simulink model "FinalModel"  (R2017b)
settings: Solver=VariableStepAuto  StartTime=0.0  StopTime=0.1  MaxStep=1e-4  RelTol=1e-3
undefined symbols (not defined in the file): D1, Delta
libraries: powerlib x31, powerlib_meascontrol x9, simulink x1, re_lib x1
settings Model: Creator=User1  LastModifiedBy=User1

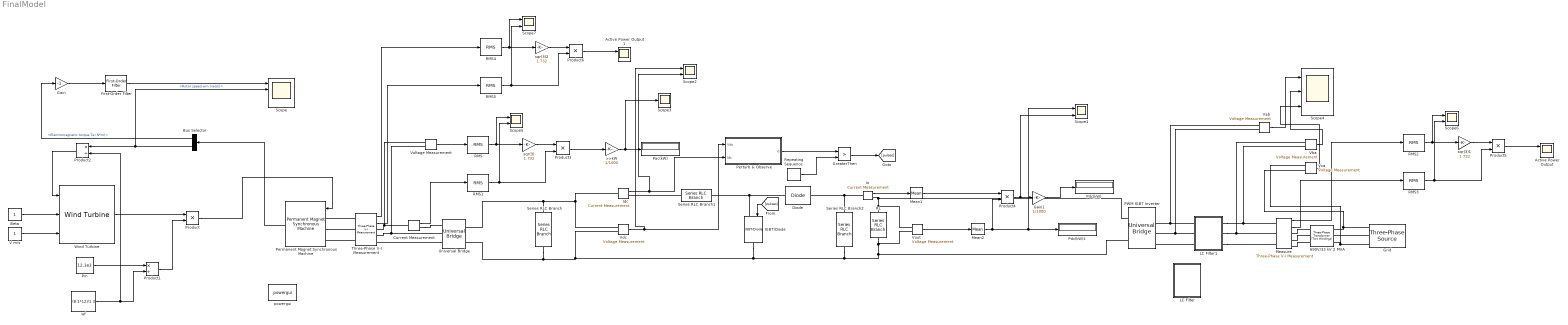
== system FinalModel ==
  690V/33 kV 2 MVA : powerlib/Elements/Three-Phase Transformer (Two Windings)  Winding1Connection=Yg  Winding2Connection=Delta (D1)  CoreType=Three single-phase transformers  SetSaturation=off  Hysteresis=off  DataFile='basic_model'  SetInitialFlux=off  Measurements=None  UNITS=SI  NominalPower=[2e6 50 ]  Winding1=[690 0.0006348 6.0619e-05]  Winding2=[33000 4.356 0.41597]  Rm=119.03  Lm=0.37887  L0=0.5  Saturation=[0 0;11.833 2.152;2366.7 2.5106]  InitialFluxes=[1.4346 -1.4346 1.2553]  MoreParameters=off  BreakLoop=off  DataType=on  TransfoNumber=0
  >>kW : Gain  Gain=1/1000
  "Active Power Output " : Scope  NumInputPorts=2
  Active Power Output 1 : Scope  NumInputPorts=2
  Beta : Constant
  Bus Selector : BusSelector  OutputSignals=Electromagnetic torque Te (N*m),Rotor speed wm (rad/s)
  Current Measurement : powerlib/Measurements/Current Measurement  PhasorSimulation=off  OutputType=Complex  PSBequivalent=0
  Diode : powerlib/Power Electronics/Diode  Ron=0.001  Lon=0  Vf=0.8  IC=0  UseSnubber=0  Rs=inf  Cs=inf  Measurements=off
  First-Order Filter : powerlib_meascontrol/Filters/First-Order Filter  FilterType=Lowpass  Tc=10e-3  Ts=50e-6  Initialize=on  Vac_Init=[0, 0, 50]  Vdc_Init=0  PlotResponse=off  FreqRange="[0,  200,  1]"
      settings: SourceProductName=Simscape Power Systems
  Gain : Gain  Gain=-1
  Gain1 : Gain  Gain=1/1000
  GreaterThen : RelationalOperator  Operator=>  OutDataTypeStr=boolean  RndMeth=Simplest
  Grid : powerlib/Electrical Sources/Three-Phase Source  InternalConnection=Yg  VoltagePhases=off  Voltage=19052  PhaseAngle=0  Voltage_phases=[25e3 25e3 25e3]/sqrt(3)  PhaseAngles_phases=[0 -120 +120]  Frequency=50  NonIdealSource=on  SpecifyImpedance=on  Resistance=0.8929  Inductance=16.58e-3  ShortCircuitLevel=2e6  BaseVoltage=33e3  XRratio=7  BusType=swing  Pref=10e3  Qref=0  Prefabc=[10e3, 10e3, 10e3]  Qrefabc=[0, 0, 0]  Qmin=-inf  Qmax=inf
  IGBT/Diode : powerlib/Power Electronics/IGBT//Diode  Ron=1e-3  Rs=1e5  Cs=inf  Measurements=off
  Idc : powerlib/Measurements/Current Measurement  PhasorSimulation=off  OutputType=Complex  PSBequivalent=0
  Io : powerlib/Measurements/Current Measurement  PhasorSimulation=off  OutputType=Complex  PSBequivalent=0
  LC Filter : Subsystem
  LC Filter1 : Subsystem
  Mean1 : powerlib_meascontrol/Measurements/Mean  Freq=60  Vinit=0  Ts=0
  Mean2 : powerlib_meascontrol/Measurements/Mean  Freq=60  Vinit=0  Ts=0
  Measure : powerlib/Measurements/Three-Phase V-I Measurement  VoltageMeasurement=phase-to-ground  SetLabelV=off  LabelV=V1  Vpu=off  VpuLL=off  CurrentMeasurement=yes  SetLabelI=off  LabelI=I1  Ipu=off  Pbase=1e3  Vbase=380  OutputType=Magnitude  PhasorSimulation=off  PSBequivalent=0
  PWM IGBT Inverter : powerlib/Power Electronics/Universal Bridge  Arms=3  SnubberResistance=5000  SnubberCapacitance=inf  Device=IGBT / Diodes  Ron=1e-3  Lon=0  ForwardVoltages="[  0.0  0.0  ]"  ForwardVoltage=.8  GTOparameters=[ 1e-6 ,1e-6 ]  IGBTparameters=[ 1e-6 , 2e-6 ]  Measurements=All voltages and currents  Measurements_2=None  converterType=Rectifier
  Pac(kW) : Display
  Pdc(kW) : Display
  Pdc(kW)1 : Display
  Permanent Magnet Synchronous Machine : powerlib/Machines/Permanent Magnet Synchronous Machine  NbPhases=3  FluxDistribution=Sinusoidal  RotorType=Salient-pole  MechanicalLoad=Torque Tm  PresetModel=No  ShowDetailedParameters=on  MeasurementBus=off  Resistance=0.00485  Inductance=8.5e-3  dqInductances=[0.295e-3,0.395e-3]  La=0.000835  MachineConstant=Voltage Constant (V_peak L-L / krpm)  Flux=0.77186  VoltageCst=700  TorqueCst=5.789  Flat=120  Mechanical=[0.00062 0.0003035 5 0]  PolePairs=5  InitialConditions=[0,0, 0,0]  InitialConditions5ph=[0 0 0 0 0 0]  TsPowergui=0  TsBlock=-1  RefAngle=90 degrees behind phase A axis (modified Park)
      settings: SourceProductName=Simscape Power Systems
  Perturb & Observe : Subsystem
  Pm : Constant  Value=12.3e3
  Product : Product  Inputs=**
  Product1 : Product  Inputs=*/
  Product2 : Product  Inputs=*/
  Product{3..6} (4 alike) : Product
  RL : powerlib/Elements/Series RLC Branch  LConnTagsString=__new0  RConnTagsString=__new0  BranchType=R  Resistance=0.2380  Inductance=1e-3  SetiL0=off  InitialCurrent=0  Capacitance=500e-6  Setx0=off  InitialVoltage=0  Measurements=None
  RMS : powerlib_meascontrol/Measurements/RMS  TrueRMS=on  Freq=50  RMSInit=650  Ts=0.1
  RMS1 : powerlib_meascontrol/Measurements/RMS  TrueRMS=on  Freq=50  RMSInit=650  Ts=0.1
  RMS{2..5} (4 alike) : powerlib_meascontrol/Measurements/RMS  TrueRMS=on  Freq=50  RMSInit=690  Ts=0.1
  Repeating Sequence : simulink/Sources/Repeating Sequence  rep_seq_t=[0 1/20000]  rep_seq_y=[0 0.9]
  Scope : Scope  NumInputPorts=4
  Scope{1..2,5..7} (5 alike) : Scope  NumInputPorts=2
  Scope3 : Scope
  Scope4 : Scope  NumInputPorts=3
  Series RLC Branch : powerlib/Elements/Series RLC Branch  LConnTagsString=__new0  RConnTagsString=__new0  BranchType=RC  Resistance=0.005  Inductance=1e-3  SetiL0=off  InitialCurrent=0  Capacitance=500e-6  Setx0=off  InitialVoltage=0  Measurements=None
  Series RLC Branch1 : powerlib/Elements/Series RLC Branch  LConnTagsString=__new0  RConnTagsString=__new0  BranchType=L  Resistance=0  Inductance=6.123e-06  SetiL0=off  InitialCurrent=0  Capacitance=1e-6  Setx0=off  InitialVoltage=0  Measurements=None
  Series RLC Branch2 : powerlib/Elements/Series RLC Branch  LConnTagsString=__new0  RConnTagsString=__new0  BranchType=RC  Resistance=0.005  Inductance=1e-3  SetiL0=off  InitialCurrent=0  Capacitance=0.0088  Setx0=off  InitialVoltage=0  Measurements=None
  Three-Phase V-I Measurement : powerlib/Measurements/Three-Phase V-I Measurement  VoltageMeasurement=phase-to-phase  SetLabelV=off  LabelV=Vabc  Vpu=off  VpuLL=off  CurrentMeasurement=yes  SetLabelI=off  LabelI=Iabc  Ipu=off  Pbase=100e6  Vbase=500e3  OutputType=Complex  PhasorSimulation=off  PSBequivalent=0
  Universal Bridge : powerlib/Power Electronics/Universal Bridge  Arms=3  SnubberResistance=1e5  SnubberCapacitance=inf  Device=Diodes  Ron=1e-3  Lon=0  ForwardVoltages="[  0  0  ]"  ForwardVoltage=0  GTOparameters=[ 10e-6 , 20e-6 ]  IGBTparameters=[ 1e-6 , 2e-6 ]  Measurements=None  Measurements_2=None  converterType=Rectifier
  V m/s : Constant
  Vab : powerlib/Measurements/Voltage Measurement  Tag=PoWeRsYsTeMmEaSuReMeNt  PhasorSimulation=off  OutputType=Magnitude  PSBequivalent=0
  Vba : powerlib/Measurements/Voltage Measurement  Tag=PoWeRsYsTeMmEaSuReMeNt  PhasorSimulation=off  OutputType=Magnitude  PSBequivalent=0
  Vca : powerlib/Measurements/Voltage Measurement  Tag=PoWeRsYsTeMmEaSuReMeNt  PhasorSimulation=off  OutputType=Magnitude  PSBequivalent=0
  Vdc : powerlib/Measurements/Voltage Measurement  PhasorSimulation=off  OutputType=Complex  PSBequivalent=0
  Voltage Measurement : powerlib/Measurements/Voltage Measurement  PhasorSimulation=off  OutputType=Complex  PSBequivalent=0
  Vout : powerlib/Measurements/Voltage Measurement  PhasorSimulation=off  OutputType=Complex  PSBequivalent=0
  Wind Turbine : re_lib/Wind Generation/Wind Turbine  Pnom=2e6  Pelec_base=8e6/0.9  wind_base=12  P_wind_base=0.73  speed_nom=1.2  pitch_angle=0  c1_c6="[0.51763          116          0.4            5           21     0.006795]"  cp_nom=0.48  lambda_nom=8.1
      settings: SourceProductName=Simscape Power Systems  SourceProductBaseCode=PS
  powergui : powerlib/powergui  Priority=1  SimulationMode=Continuous  SampleTime=1e-6  frequency=60  Iterations=50  frequencyindice=0  Pbase=100e6  ErrMax=1e-4  UnitsV=kV  UnitsW=MW  buscounter=0  FunctionMessages=off  echomessages=off  EnableUseOfTLC=off  CurrentSourceSwitches=off  DisableSnubberDevices=off  DisableRonSwitches=off  DisableVfSwitches=off  DisplayEquations=off  SolverType=Tustin/Backward Euler (TBE)  Interpol=off  ExternalGateDelay=off  methode=off  Ts=100  x0status=blocks  SPID=on  SwTol=0  HookPort=off  RestoreLinks=warning  ResistiveCurrentMeasurement=off  Frange=[0:2:500]  Ylog=off  Xlog=on  ShowGrid=off  save=off  variable=ZData  structure=0  ZoomFFT=off  StartTime=0.0  cycles=1  DisplayStyle=1  fundamental=60  FreqAxis=off  MaxFrequency=1000  frequencyindicesteady=1  RmsSteady=1  display=off
  sqr(3) : Gain  Gain=1.732
  sqr(3)1 : Gain  Gain=1.732
  sqr(3)2 : Gain  Gain=1.732
  wf : Constant  Value=(8.1*12)/1.3
  wires:
  Wind Turbine/1 -> Product/1
  Pm/1 -> Product1/1
  wf/1 -> Product2/2, Product1/2
  Product1/1 -> Product/2
  Product/1 -> Permanent Magnet Synchronous Machine/1
  Permanent Magnet Synchronous Machine/1 -> Bus Selector/1
  Bus Selector/1 -> Gain/1  "<Electromagnetic torque Te (N*m)>"
  Bus Selector/2 -> Scope/2, Product2/1  "<Rotor speed wm (rad/s)>"
  V m/s/1 -> Wind Turbine/3
  Beta/1 -> Wind Turbine/2
  Product2/1 -> Wind Turbine/1
  First-Order Filter/1 -> Scope/1
  Gain/1 -> First-Order Filter/1
  Voltage Measurement/1 -> RMS/1
  Current Measurement/1 -> RMS1/1
  RMS/1 -> Scope5/1, sqr(3)/1
  RMS1/1 -> Scope5/2, Product3/2
  sqr(3)/1 -> Product3/1
  Product3/1 -> >>kW/1
  >>kW/1 -> Scope3/1, Pac(kW)/1
  Vdc/1 -> Scope2/1, Perturb & Observe/1("Vdc ")
  Idc/1 -> Scope2/2, Perturb & Observe/2("Idc ")
  Perturb & Observe/1(d) -> GreaterThen/1
  Repeating Sequence/1 -> GreaterThen/2
  GreaterThen/1 -> [pulses]
  [pulses] -> IGBT/Diode/1
  Io/1 -> Mean1/1
  Vout/1 -> Mean2/1
  Mean1/1 -> Product4/1
  Gain1/1 -> Pdc(kW)/1
  Vba/1 -> Scope4/2
  Vab/1 -> Scope4/1
  Vca/1 -> Scope4/3
  Mean2/1 -> Scope1/1, Pdc(kW)1/1, Product4/2
  Product4/1 -> Scope1/2, Gain1/1
  sqr(3)1/1 -> Product5/1
  Measure/1 -> RMS2/1
  Measure/2 -> RMS3/1
  RMS3/1 -> Scope6/2, Product5/2
  RMS2/1 -> Scope6/1, sqr(3)1/1
  Product5/1 -> "Active Power Output "/1
  RMS5/1 -> Scope7/2, Product6/2
  RMS4/1 -> Scope7/1, sqr(3)2/1
  Three-Phase V-I Measurement/1 -> RMS4/1
  Three-Phase V-I Measurement/2 -> RMS5/1
  Product6/1 -> Active Power Output 1/1
  sqr(3)2/1 -> Product6/1
  connections:
  Three-Phase V-I Measurement/LConn1 -- Permanent Magnet Synchronous Machine/LConn1
  Three-Phase V-I Measurement/LConn2 -- Permanent Magnet Synchronous Machine/LConn2
  Three-Phase V-I Measurement/LConn3 -- Permanent Magnet Synchronous Machine/LConn3
  Voltage Measurement/LConn1 -- Current Measurement/LConn1 -- Three-Phase V-I Measurement/RConn1
  Universal Bridge/LConn2 -- Voltage Measurement/LConn2 -- Three-Phase V-I Measurement/RConn2
  Universal Bridge/LConn3 -- Three-Phase V-I Measurement/RConn3
  Current Measurement/RConn1 -- Universal Bridge/LConn1
  Series RLC Branch/LConn1 -- Vdc/LConn1 -- Idc/LConn1 -- Universal Bridge/RConn1
  Series RLC Branch/RConn1 -- PWM IGBT Inverter/RConn2 -- Vout/LConn2 -- RL/RConn1 -- Series RLC Branch2/RConn1 -- IGBT/Diode/RConn1 -- Vdc/LConn2 -- Universal Bridge/RConn2
  Series RLC Branch1/LConn1 -- Idc/RConn1
  IGBT/Diode/LConn1 -- Diode/LConn1 -- Series RLC Branch1/RConn1
  RL/LConn1 -- PWM IGBT Inverter/RConn1 -- Io/RConn1 -- Vout/LConn1
  Series RLC Branch2/LConn1 -- Io/LConn1 -- Diode/RConn1
  Vba/LConn2 -- Measure/LConn1 -- LC Filter1/RConn1
  Vba/LConn1 -- LC Filter1/RConn2 -- Measure/LConn2
  Measure/RConn1 -- 690V/33 kV 2 MVA/LConn1
  Measure/RConn2 -- 690V/33 kV 2 MVA/LConn2
  Measure/RConn3 -- 690V/33 kV 2 MVA/LConn3
  Grid/RConn1 -- Vca/LConn2 -- 690V/33 kV 2 MVA/RConn1
  Grid/RConn2 -- 690V/33 kV 2 MVA/RConn2
  Grid/RConn3 -- Vca/LConn1 -- 690V/33 kV 2 MVA/RConn3
  Vab/LConn1 -- LC Filter1/LConn1 -- PWM IGBT Inverter/LConn1
  Vab/LConn2 -- LC Filter1/LConn2 -- PWM IGBT Inverter/LConn2
  LC Filter1/LConn3 -- PWM IGBT Inverter/LConn3
  LC Filter1/RConn3 -- Measure/LConn3

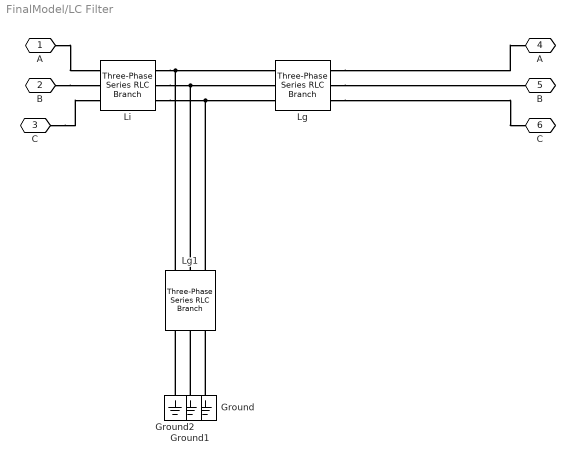
== system FinalModel/LC Filter ==
  Ground : powerlib/Elements/Ground  LConnTagsString=a
  Ground1 : powerlib/Elements/Ground  LConnTagsString=a
  Ground2 : powerlib/Elements/Ground  LConnTagsString=a
  Lg : powerlib/Elements/Three-Phase Series RLC Branch  LConnTagsString=A|B|C  RConnTagsString=A|B|C  BranchType=RL  Resistance=267.81  Inductance=0.0030  Capacitance=inf  Measurements=Branch voltages and currents
  Lg1 : powerlib/Elements/Three-Phase Series RLC Branch  LConnTagsString=A|B|C  RConnTagsString=A|B|C  BranchType=RC  Resistance=267.81  Inductance=2e-3  Capacitance=2.9239e-09  Measurements=Branch voltages and currents
  "Li " : powerlib/Elements/Three-Phase Series RLC Branch  LConnTagsString=A|B|C  RConnTagsString=A|B|C  BranchType=RL  Resistance=267.81  Inductance=0.0050  Capacitance=inf  Measurements=Branch voltages and currents
  A : PMIOPort  Port=1  Side=Left
  B : PMIOPort  Port=2  Side=Left
  C : PMIOPort  Port=3  Side=Left
  "A " : PMIOPort  Port=4  Side=Right
  "B " : PMIOPort  Port=5  Side=Right
  "C " : PMIOPort  Port=6  Side=Right
  connections:
  B/RConn1 -- "Li "/LConn2
  A/RConn1 -- "Li "/LConn1
  C/RConn1 -- "Li "/LConn3
  Lg/RConn1 -- "A "/RConn1
  "Li "/RConn2 -- Lg1/LConn2 -- Lg/LConn2
  "Li "/RConn3 -- Lg1/LConn3 -- Lg/LConn3
  Lg/RConn3 -- "C "/RConn1
  Lg/RConn2 -- "B "/RConn1
  "Li "/RConn1 -- Lg1/LConn1 -- Lg/LConn1
  Ground/LConn1 -- Lg1/RConn3
  Ground1/LConn1 -- Lg1/RConn2
  Ground2/LConn1 -- Lg1/RConn1

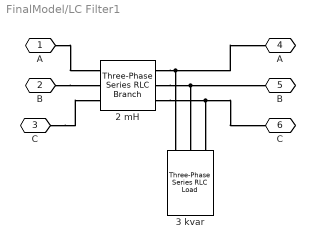
== system FinalModel/LC Filter1 ==
  "2 mH " : powerlib/Elements/Three-Phase Series RLC Branch  LConnTagsString=A|B|C  RConnTagsString=A|B|C  BranchType=L  Resistance=0  Inductance=2e-3  Capacitance=inf  Measurements=Branch voltages and currents
  3 kvar : powerlib/Elements/Three-Phase Series RLC Load  LConnTagsString=A|B|C  Configuration=Y (grounded)  NominalVoltage=690  Vabc=[1e3 1e3 1e3]  Vabcp=[1e3 1e3 1e3]  NominalFrequency=50  UnbalancedPower=off  ActivePower=0  InductivePower=0  CapacitivePower=10e3  Pabc=[10e3 9e3 11e3]  QLabc=[100 90 110]  QCabc=[100 90 110]  Pabcp=[10e3 9e3 11e3]  QLabcp=[100 90 110]  QCabcp=[100 90 110]  Measurements=None  LoadType=constant Z
  A : PMIOPort  Port=1  Side=Left
  B : PMIOPort  Port=2  Side=Left
  C : PMIOPort  Port=3  Side=Left
  "A " : PMIOPort  Port=4  Side=Right
  "B " : PMIOPort  Port=5  Side=Right
  "C " : PMIOPort  Port=6  Side=Right
  connections:
  B/RConn1 -- "2 mH "/LConn2
  A/RConn1 -- "2 mH "/LConn1
  C/RConn1 -- "2 mH "/LConn3
  "2 mH "/RConn1 -- "A "/RConn1 -- 3 kvar/LConn1
  "2 mH "/RConn2 -- "B "/RConn1 -- 3 kvar/LConn2
  "2 mH "/RConn3 -- "C "/RConn1 -- 3 kvar/LConn3

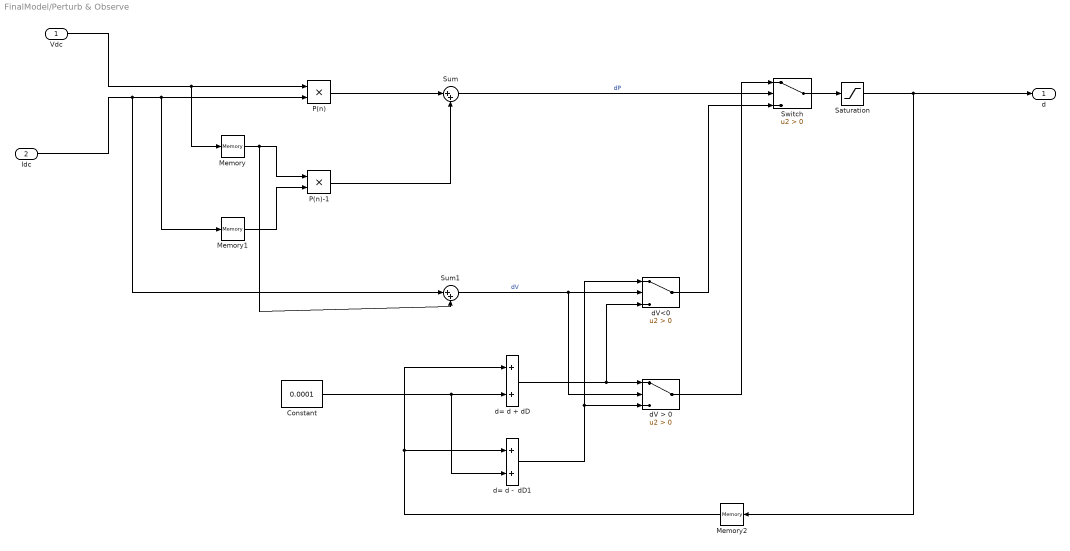
== system FinalModel/Perturb & Observe ==
  "Vdc " : Inport
  "Idc " : Inport  Port=2
  Constant : Constant  Value=0.0001
  Memory : Memory
  Memory1 : Memory
  Memory2 : Memory
  P(n) : Product
  P(n)-1 : Product
  Saturation : Saturate  UpperLimit=inf
  Sum : Sum  Inputs=|++
  Sum1 : Sum  Inputs=|++
  Switch : Switch  Criteria=u2 > Threshold
  d= d + dD : Sum
  d= d -  dD1 : Sum
  dV > 0 : Switch  Criteria=u2 > Threshold
  dV<0 : Switch  Criteria=u2 > Threshold
  d : Outport
  wires:
  "Vdc "/1 -> Memory/1, P(n)/1
  "Idc "/1 -> Sum1/1, Memory1/1, P(n)/2
  Memory/1 -> Sum1/2, P(n)-1/1
  Memory1/1 -> P(n)-1/2
  P(n)/1 -> Sum/1
  P(n)-1/1 -> Sum/2
  Sum/1 -> Switch/2  "dP"
  Sum1/1 -> dV > 0/2, dV<0/2  "dV"
  Switch/1 -> Saturation/1
  Memory2/1 -> d= d -  dD1/1, d= d + dD/1
  Constant/1 -> d= d -  dD1/2, d= d + dD/2
  d= d -  dD1/1 -> dV<0/1, dV > 0/3
  d= d + dD/1 -> dV<0/3, dV > 0/1
  dV<0/1 -> Switch/3
  dV > 0/1 -> Switch/1
  Saturation/1 -> Memory2/1, d/1
